simulink model "Q_4"  (R2016b)
settings: Solver=VariableStepAuto  StartTime=0.0  StopTime=totaltime  RelTol=1e-3
values from neighbouring files (symbols this model uses):
  N = NN    (= 1024)    [IIR_Response.m]    (also in lab2_Q3.m = 40000)
  st = 1/1e5    (= 1e-05)    [IIR_Response.m]    (also in lab2_Q3.m)
  st2 = st/2    (= 5e-06)    [IIR_Response.m]
undefined symbols (not defined in the file or in its folder): A
libraries: xbsIndex_r4 x4, JTAGRuntimeCosim_r4 x1
settings Model: Creator=rm101  LastModifiedBy=rm101

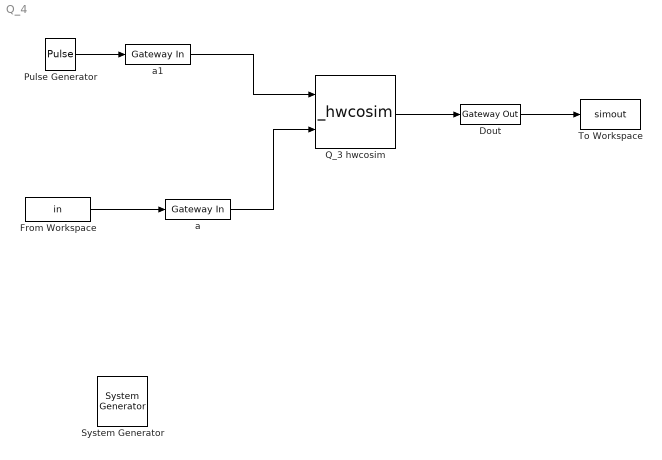
== system Q_4 ==
  " System Generator" : xbsIndex_r4/ System Generator  Tag=genX  xilinxfamily=zynq  part=xc7z020  speed=-1  package=clg484  synthesis_tool=Vivado  clock_wrapper=Clock Enables  directory=E:/YG/generator/5_3  proj_type=Vivado  Synth_file=Vivado Synthesis Defaults  Impl_file=Vivado Implementation Defaults  testbench=off  simulink_period=st2  sysclk_period=st2*10e8  dcm_input_clock_period=10  incr_netlist=off  trim_vbits=Everywhere in SubSystem  dbl_ovrd=According to Block Masks  core_generation=According to Block Masks  run_coregen=off  deprecated_control=off  eval_field=0  block_type=sysgen
  Dout : xbsIndex_r4/Gateway Out  inherit_from_input=off  hdl_port=on  rows=1  columns=1  UseAsDAC=off  DACChannel='1'  interface=None  automatic_assignment=on  address_offset=hex2dec('00')  intf_name=''  intf_description=''  timing_constraint=None  locs_specified=off  LOCs={}  io_standard={}  block_type=gatewayout
  From Workspace : FromWorkspace  VariableName=in  SampleTime=0  Interpolate=off  OutputAfterFinalValue=Holding final value
  Pulse Generator : DiscretePulseGenerator  PulseType=Time based  Period=st  PulseWidth=50
  Q_3 hwcosim : JTAGRuntimeCosim_r4/_hwcosim  clkSrc=Single Stepped  hasCombinationalPath=on  bitfileName=E:\YG\generator\5_3\q_3.bit  skipConfig=off  dispPartInfo=off  useZynqReconfigScript=on  cable=Auto Detect  speed=N/A  cablePort=N/A  cableLocation=Local  shareCable=off  design_xtable=|  engineDll=JTAGCosimEngine.dll  cableWaitTime=10  bscanPos=-1  IRLengths=[]  useWaitBox=1  hasBufgmux=on  Scheme=Cosim  useCmdProc=1  hasProc=0  useImpact=0  printLogFile=0  userChain=2  block_type=jtagcosim
      | {
      |     'clkWrapper' => 'q_3',
      |     'burstMode' => false,
      |     'burstFifoDepth' => '1024',
      |     'shared_memories' => {},
      |     'clocksGcd' => 1,
      |     'device' => {
      |       'family' => 'zynq',
      |       'part' => 'xc7z020',
      |       'package' => 'clg484',
      |       'speed' => '-1',
      |     },
      |     'ports' => {
      |       'a1' => {
      |         'direction' => 'in',
      |         'width' => 1,
      |         'name' => 'a1',
      |         'period' => 1,
      |         'icon_text' => 'a1',
      |         'type' => 'Bool',
      |         'arithmetic_type' => 'xlUnsigned',
      |         'dat_file' => 'q_3_a1.dat',
      |         'bin_pt' => 0,
      |         'addr_offset' => 0,
      |         'bd_port_index' => 0,
      |       },
      |       'a' => {
      |         'direction' => 'in',
      |         'width' => 8,
      |         'name' => 'a',
      |         'period' => 2,
      |         'icon_text' => 'a',
      |         'type' => 'Fix_8_6',
      |         'arithmetic_type' => 'xlSigned',
      |         'dat_file' => 'q_3_a.dat',
      |         'bin_pt' => 6,
      |         'addr_offset' => 4,
      |         'bd_port_index' => 1,
      |       },
      |       'dout' => {
      |         'direction' => 'out',
      |         'width' => 17,
      |         'name' => 'dout',
      |         'period' => 2,
      |         'icon_text' => 'Dout',
      |         'type' => 'Fix_17_14',
      |         'arithmetic_type' => 'xlSigned',
      |         'dat_file' => 'q_3_dout.dat',
      |         'bin_pt' => 14,
      |         'addr_offset' => 8,
      |         'bd_port_index' => 0,
      |       },
      |     },
      |   }
  To Workspace : ToWorkspace  VariableName=simout  SaveFormat=Timeseries  SampleTime=-1
  a : xbsIndex_r4/Gateway In  gui_display_data_type=Fixed-point  arith_type="Signed  (2's comp)"  n_bits=8  bin_pt=6  preci_type=Single  exp_width=8  frac_width=24  rows=1  columns=1  quantization="Round  (unbiased: +/- Inf)"  overflow=Saturate  period=st  UseAsADC=off  ADCChannel='1'  interface=None  automatic_assignment=on  address_offset=hex2dec('00')  intf_name=''  intf_description=''  default_value=0  timing_constraint=None  locs_specified=off  LOCs={}  io_standard={}  inherit_from_input=off  hdl_port=on  dbl_ovrd=off  block_type=gatewayin
  a1 : xbsIndex_r4/Gateway In  gui_display_data_type=Boolean  arith_type=Boolean  n_bits=1  bin_pt=0  preci_type=Single  exp_width=8  frac_width=24  rows=1  columns=1  quantization="Round  (unbiased: +/- Inf)"  overflow=Saturate  period=st2  UseAsADC=off  ADCChannel='1'  interface=None  automatic_assignment=on  address_offset=hex2dec('00')  intf_name=''  intf_description=''  default_value=0  timing_constraint=None  locs_specified=off  LOCs={}  io_standard={}  inherit_from_input=off  hdl_port=on  dbl_ovrd=off  block_type=gatewayin
  wires:
  From Workspace/1 -> a/1
  Pulse Generator/1 -> a1/1
  Dout/1 -> To Workspace/1
  Q_3 hwcosim/1 -> Dout/1
  a1/1 -> Q_3 hwcosim/1
  a/1 -> Q_3 hwcosim/2
